simulink model "gm_am_demod_hdl_coder_vnl"  (R2021b)
settings: Solver=FixedStepAuto  StartTime=0.0  StopTime=20  RelTol=1e-3  EnableMultiTasking=on
libraries: hdlmdlgenlib x10, simulink x1
settings Model: Creator=caccolillo  LastModifiedBy=caccolillo
settings SolverCC: AutoInsertRateTranBlk=on
settings OptimizationCC: BlockReduction=off  ConditionallyExecuteInputs=off  DefaultParameterBehavior=Inlined  UseDivisionForNetSlopeComputation=on  GainParamInheritBuiltInType=on  UseFloatMulNetSlope=on  InlineInvariantSignals=on  EfficientFloat2IntCast=on  LifeSpan=1
settings DebuggingCC: AlgebraicLoopMsg=error  InheritedTsInSrcMsg=none  SingleTaskRateTransMsg=error
settings HardwareCC: ProdBitPerPointer=32  ProdBitPerSizeT=32  ProdBitPerPtrDiffT=32  ProdLargestAtomicFloat=None  ProdIntDivRoundTo=Undefined  ProdEndianess=Unspecified  ProdWordSize=32  ProdHWDeviceType=ASIC/FPGA->ASIC/FPGA  TargetBitPerLong=64  TargetBitPerPointer=64  TargetBitPerSizeT=64  TargetBitPerPtrDiffT=64  TargetLongLongMode=on  TargetIntDivRoundTo=Zero  TargetEndianess=LittleEndian  TargetWordSize=64  TargetHWDeviceType=Custom Processor->MATLAB Host Computer  ProdEqTarget=off
settings SFSimCC: MATLABDynamicMemAlloc=off
settings RTWCC: GenerateReport=on  LaunchReport=on
settings CodeAppCC: ForceParamTrailComments=on
settings GRTTargetCC: CombineSignalStateStructs=on  MatFileLogging=off  SupportVariableSizeSignals=on

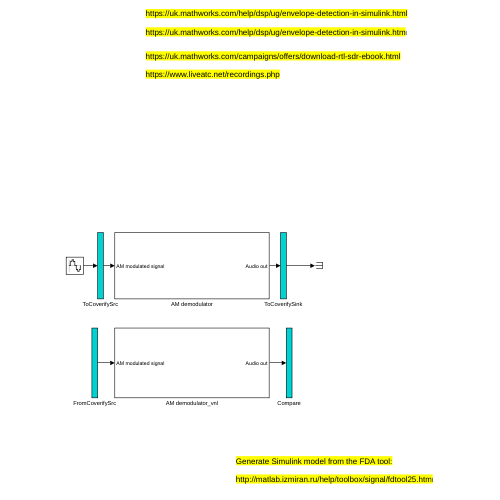
[thumbnail: Simulink's stored preview of the top-level diagram]
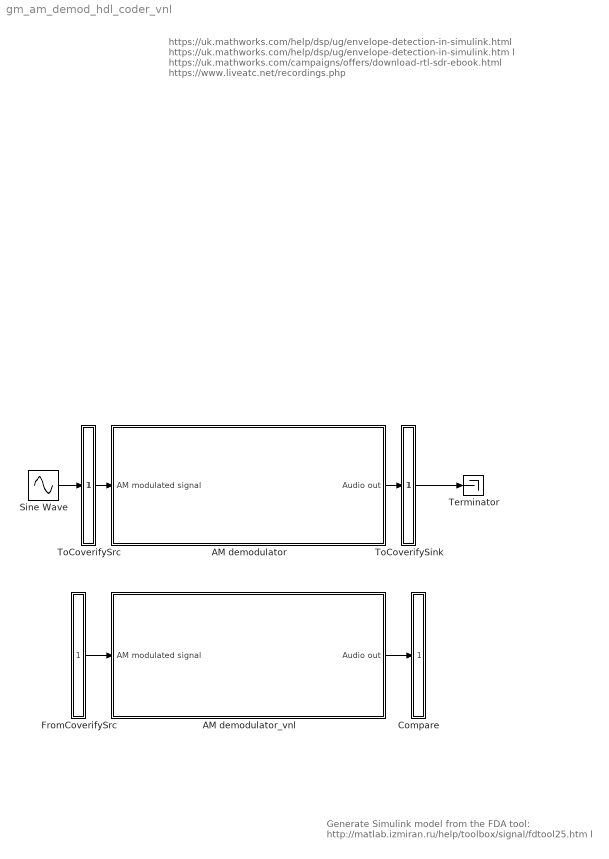
== system gm_am_demod_hdl_coder_vnl ==
  note: Generate Simulink model from the FDA tool:
      |
      | http://matlab.izmiran.ru/help/toolbox/signal/fdtool25.htm l
  note: https://uk.mathworks.com/help/dsp/ug/envelope-detection-in-simulink.html
      |
      | https://uk.mathworks.com/help/dsp/ug/envelope-detection-in-simulink.htm l
      |
      | https://uk.mathworks.com/campaigns/offers/download-rtl-sdr-ebook.html
      |
      | https://www.liveatc.net/recordings.php
  AM demodulator : Subsystem
  AM demodulator_vnl : Subsystem
  Compare : Subsystem
      mask Display: disp('')
  FromCoverifySrc : Subsystem
      mask Display: disp('')
  Sine Wave : Sin  SampleTime=1e-6
  Terminator : Terminator
  ToCoverifySink : Subsystem
      mask Display: disp('')
  ToCoverifySrc : Subsystem
      mask Display: disp('')
  wires:
  ToCoverifySrc/1(out1) -> AM demodulator/1(AM modulated signal)
  AM demodulator/1(Audio out) -> ToCoverifySink/1(in1)
  Sine Wave/1 -> ToCoverifySrc/1(in1)
  ToCoverifySink/1(out1) -> Terminator/1
  FromCoverifySrc/1(out1) -> AM demodulator_vnl/1(AM modulated signal)
  AM demodulator_vnl/1(Audio out) -> Compare/1(in1)

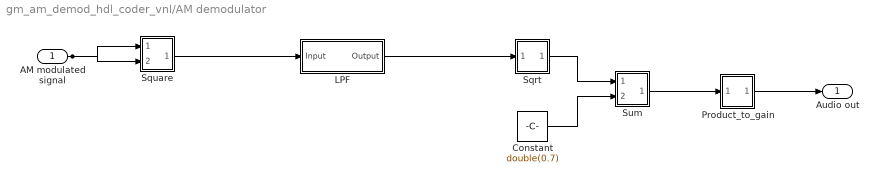
== system gm_am_demod_hdl_coder_vnl/AM demodulator ==
  AM modulated signal : Inport  OutDataTypeStr=double  PortDimensions=1  SampleTime=1e-06
  Constant : Constant  Value=double(0.7)  OutDataTypeStr=double  SampleTime=1e-06
  LPF : Subsystem
  Product_to_gain : Subsystem
      mask Display: disp('NFP\ngain_pow2');
  Sqrt : Subsystem
      mask Display: disp('NFP\nsqrt');
  Square : Subsystem
      mask Display: disp('NFP\nmul');
  Sum : Subsystem
      mask Display: disp('NFP\nadd');
  Audio out : Outport  SampleTime=1e-06
  wires:
  Product_to_gain/1(Out1) -> Audio out/1
  Sum/1(Out1) -> Product_to_gain/1(In1)
  Square/1(Out1) -> LPF/1(Input)
  Sqrt/1(Out1) -> Sum/1(In1)
  LPF/1(Output) -> Sqrt/1(In1)
  Constant/1 -> Sum/2(In2)
  AM modulated signal/1 -> Square/1(In1), Square/2(In2)

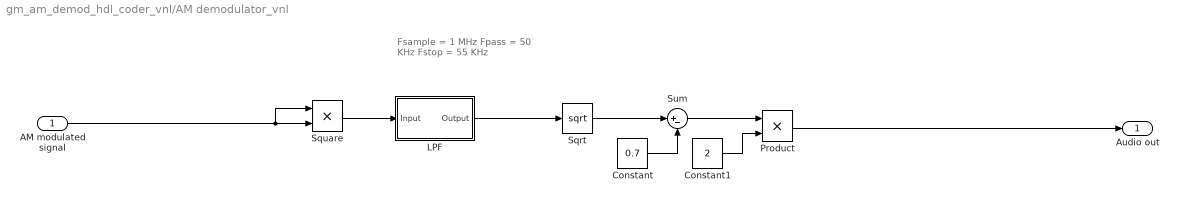
== system gm_am_demod_hdl_coder_vnl/AM demodulator_vnl ==
  note: Fsample = 1 MHz
      | Fpass =  50 KHz
      | Fstop =  55 KHz
  AM modulated signal : Inport  SampleTime=1e-6
  Constant : Constant  Value=0.7  SampleTime=1e-6
  Constant1 : Constant  Value=2  SampleTime=1e-6
  LPF : Subsystem  Tag=FilterWizardSubSystem
      settings: ErrorFcn=dspFilterRealizedInBasicElemsAlgLoopErrFcnCallback
  Product : Product
  Sqrt : Sqrt  SaturateOnIntegerOverflow=on
  Square : Product
  Sum : Sum  Inputs=|+-
  Audio out : Outport
  wires:
  Product/1 -> Audio out/1
  LPF/1(Output) -> Sqrt/1
  Constant1/1 -> Product/2
  Sum/1 -> Product/1
  Constant/1 -> Sum/2
  AM modulated signal/1 -> Square/2, Square/1
  Sqrt/1 -> Sum/1
  Square/1 -> LPF/1(Input)

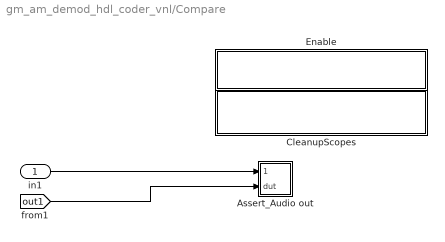
== system gm_am_demod_hdl_coder_vnl/Compare ==
  in1 : Inport
  Assert_Audio out : Subsystem  mask{ToleranceValue=1e-07}
  CleanupScopes : Subsystem
      settings: OpenFcn=|
      | blkName = gcb; %self block
      | idx = regexp(blkName, '/CleanupScopes$', 'once');
      | blkParent = blkName(1:idx-1);
      | blks=find_system(blkParent, 'LookUnderMasks', 'all','blocktype', 'Scope');
      | for itr = 1:length(blks)
      | 	 hScopeCfg = get_param(blks{itr},'ScopeConfiguration');
      | 	 hScopeCfg.Visible = ~ hScopeCfg.Visible;
      | end
      | drawnow;
      mask Display: fprintf(message('hdlcoder:cosim:vnl_dblclick').getString());
  Enable : Subsystem
      settings: OpenFcn=|
      | blkName = gcb;
      | idx = regexp(blkName, '/Enable$', 'once');
      | blkParent = blkName(1:idx-1);
      | blks=find_system(blkParent, 'LookUnderMasks', 'all','blocktype', 'Assertion');
      | e = get_param(blks{1}, 'Enabled');
      | if strcmp(e, 'on'), f= 'off';, else, f = 'on';, end
      | for ii=1:length(blks), set_param(blks{ii}, 'Enabled', f);, end
      | set_param(gcb, 'MaskDisplay',['fprintf(message(''hdlcoder:cosim:vnl_dblclick_assertions'',','''',upper(e),'''',').getString())']);
      mask Display: fprintf(message('hdlcoder:cosim:vnl_dblclick_assertions','OFF').getString());
  wires:
  in1/1 -> Assert_Audio out/1(cosim)
  [out1] -> Assert_Audio out/2(dut)

== system gm_am_demod_hdl_coder_vnl/FromCoverifySrc ==
  out1 : Outport
  wires:
  [in1] -> out1/1

== system gm_am_demod_hdl_coder_vnl/ToCoverifySink ==
  in1 : Inport
  out1 : Outport
  tag scope: out1=global
  wires:
  in1/1 -> out1/1, [out1]

== system gm_am_demod_hdl_coder_vnl/ToCoverifySrc ==
  in1 : Inport
  out1 : Outport
  tag scope: in1=global
  wires:
  in1/1 -> out1/1, [in1]

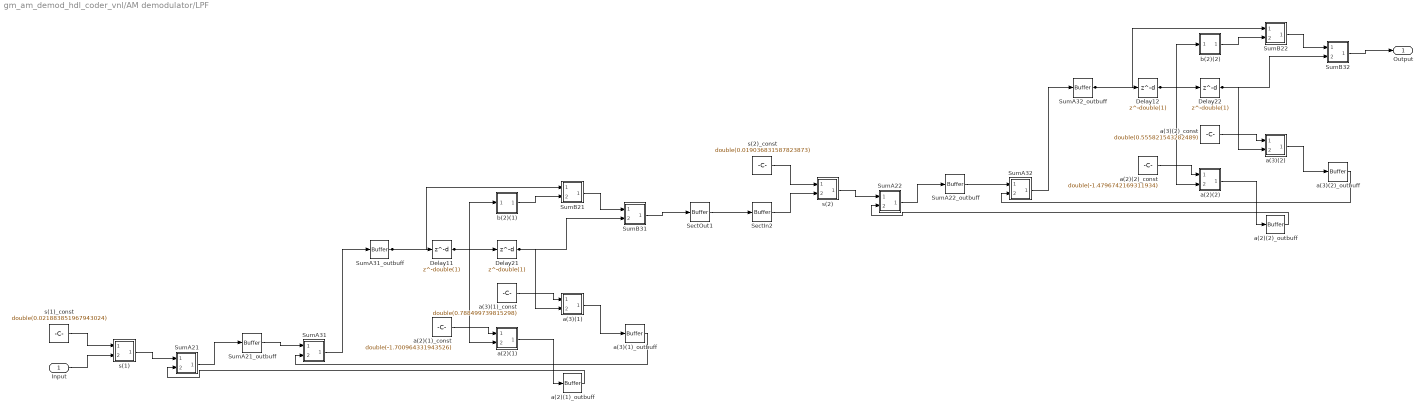
== system gm_am_demod_hdl_coder_vnl/AM demodulator/LPF ==
  Input : Inport  OutDataTypeStr=double  PortDimensions=1  SampleTime=1e-06
  Delay{11..12,21..22} (4 alike) : Delay  DelayLength=double(1)  InitialCondition=0  SampleTime=1e-06
  SectIn2 : hdlmdlgenlib/Buffer
      settings: SourceProductBaseCode=SL
  SectOut1 : hdlmdlgenlib/Buffer
      settings: SourceProductBaseCode=SL
  SumA21 : Subsystem
      mask Display: disp('NFP\nadd');
  SumA21_outbuff : hdlmdlgenlib/Buffer
      settings: SourceProductBaseCode=SL
  SumA22 : Subsystem
      mask Display: disp('NFP\nadd');
  SumA22_outbuff : hdlmdlgenlib/Buffer
      settings: SourceProductBaseCode=SL
  SumA31 : Subsystem
      mask Display: disp('NFP\nadd');
  SumA31_outbuff : hdlmdlgenlib/Buffer
      settings: SourceProductBaseCode=SL
  SumA32 : Subsystem
      mask Display: disp('NFP\nadd');
  SumA32_outbuff : hdlmdlgenlib/Buffer
      settings: SourceProductBaseCode=SL
  SumB21 : Subsystem
      mask Display: disp('NFP\nadd');
  SumB22 : Subsystem
      mask Display: disp('NFP\nadd');
  SumB31 : Subsystem
      mask Display: disp('NFP\nadd');
  SumB32 : Subsystem
      mask Display: disp('NFP\nadd');
  a(2)(1) : Subsystem
      mask Display: disp('NFP\nmul');
  a(2)(1)_const : Constant  Value=double(-1.700964331943526)  OutDataTypeStr=double  SampleTime=1e-06
  a(2)(1)_outbuff : hdlmdlgenlib/Buffer
      settings: SourceProductBaseCode=SL
  a(2)(2) : Subsystem
      mask Display: disp('NFP\nmul');
  a(2)(2)_const : Constant  Value=double(-1.4796742169311934)  OutDataTypeStr=double  SampleTime=1e-06
  a(2)(2)_outbuff : hdlmdlgenlib/Buffer
      settings: SourceProductBaseCode=SL
  a(3)(1) : Subsystem
      mask Display: disp('NFP\nmul');
  a(3)(1)_const : Constant  Value=double(0.788499739815298)  OutDataTypeStr=double  SampleTime=1e-06
  a(3)(1)_outbuff : hdlmdlgenlib/Buffer
      settings: SourceProductBaseCode=SL
  a(3)(2) : Subsystem
      mask Display: disp('NFP\nmul');
  a(3)(2)_const : Constant  Value=double(0.555821543282489)  OutDataTypeStr=double  SampleTime=1e-06
  a(3)(2)_outbuff : hdlmdlgenlib/Buffer
      settings: SourceProductBaseCode=SL
  b(2)(1) : Subsystem
      mask Display: disp('NFP\ngain_pow2');
  b(2)(2) : Subsystem
      mask Display: disp('NFP\ngain_pow2');
  s(1) : Subsystem
      mask Display: disp('NFP\nmul');
  s(1)_const : Constant  Value=double(0.021883851967943024)  OutDataTypeStr=double  SampleTime=1e-06
  s(2) : Subsystem
      mask Display: disp('NFP\nmul');
  s(2)_const : Constant  Value=double(0.019036831587823873)  OutDataTypeStr=double  SampleTime=1e-06
  Output : Outport  SampleTime=1e-06
  wires:
  s(2)/1(Out1) -> SumA22/1(In1)
  s(1)/1(Out1) -> SumA21/1(In1)
  a(3)(2)/1(Out1) -> a(3)(2)_outbuff/1
  a(3)(1)/1(Out1) -> a(3)(1)_outbuff/1
  a(2)(2)/1(Out1) -> a(2)(2)_outbuff/1
  a(2)(1)/1(Out1) -> a(2)(1)_outbuff/1
  SumB32/1(Out1) -> Output/1
  SumB31/1(Out1) -> SectOut1/1
  SumB22/1(Out1) -> SumB32/1(In1)
  SumB21/1(Out1) -> SumB31/1(In1)
  SumA32/1(Out1) -> SumA32_outbuff/1
  SumA31/1(Out1) -> SumA31_outbuff/1
  SumA22/1(Out1) -> SumA22_outbuff/1
  SumA21/1(Out1) -> SumA21_outbuff/1
  b(2)(2)/1(Out1) -> SumB22/2(In2)
  b(2)(1)/1(Out1) -> SumB21/2(In2)
  s(2)_const/1 -> s(2)/1(In1)
  s(1)_const/1 -> s(1)/1(In1)
  a(3)(2)_const/1 -> a(3)(2)/1(In1)
  a(3)(1)_const/1 -> a(3)(1)/1(In1)
  a(2)(2)_const/1 -> a(2)(2)/1(In1)
  a(2)(1)_const/1 -> a(2)(1)/1(In1)
  SectOut1/1 -> SectIn2/1
  a(3)(2)_outbuff/1 -> SumA32/2(In2)
  a(3)(1)_outbuff/1 -> SumA31/2(In2)
  a(2)(2)_outbuff/1 -> SumA22/2(In2)
  a(2)(1)_outbuff/1 -> SumA21/2(In2)
  SumA32_outbuff/1 -> Delay12/1, SumB22/1(In1)
  SumA31_outbuff/1 -> Delay11/1, SumB21/1(In1)
  SumA22_outbuff/1 -> SumA32/1(In1)
  SumA21_outbuff/1 -> SumA31/1(In1)
  SectIn2/1 -> s(2)/2(In2)
  Delay22/1 -> SumB32/2(In2), a(3)(2)/2(In2)
  Delay21/1 -> SumB31/2(In2), a(3)(1)/2(In2)
  Delay12/1 -> Delay22/1, b(2)(2)/1(In1), a(2)(2)/2(In2)
  Delay11/1 -> Delay21/1, b(2)(1)/1(In1), a(2)(1)/2(In2)
  Input/1 -> s(1)/2(In2)

== system gm_am_demod_hdl_coder_vnl/AM demodulator/Product_to_gain ==
  In1 : Inport
  Product_to_gain : Gain  Gain=double(2)
  Out1 : Outport
  wires:
  Product_to_gain/1 -> Out1/1
  In1/1 -> Product_to_gain/1

== system gm_am_demod_hdl_coder_vnl/AM demodulator/Sqrt ==
  In1 : Inport
  Sqrt : Sqrt  SampleTime=1e-06  SaturateOnIntegerOverflow=on
  Out1 : Outport
  wires:
  Sqrt/1 -> Out1/1
  In1/1 -> Sqrt/1

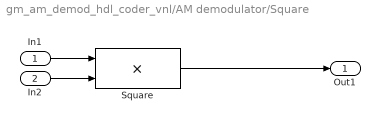
== system gm_am_demod_hdl_coder_vnl/AM demodulator/Square ==
  In1 : Inport
  In2 : Inport  Port=2
  Square : Product  Inputs=**  OutDataTypeStr=double  SampleTime=1e-06
  Out1 : Outport
  wires:
  Square/1 -> Out1/1
  In2/1 -> Square/2
  In1/1 -> Square/1

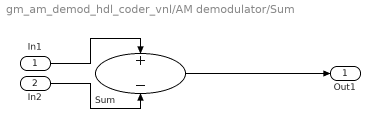
== system gm_am_demod_hdl_coder_vnl/AM demodulator/Sum ==
  In1 : Inport
  In2 : Inport  Port=2
  Sum : Sum  Inputs=+-  OutDataTypeStr=double  SampleTime=1e-06
  Out1 : Outport
  wires:
  Sum/1 -> Out1/1
  In2/1 -> Sum/2
  In1/1 -> Sum/1

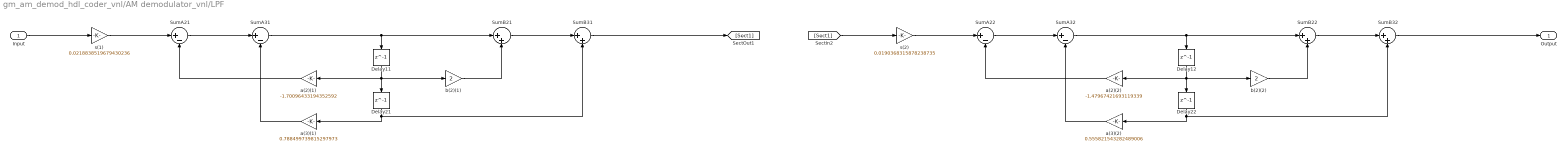
== system gm_am_demod_hdl_coder_vnl/AM demodulator_vnl/LPF ==
  Input : Inport
  Delay{11..12,21..22} (4 alike) : Delay  DelayLength=1  InitialCondition=0
  SumA{21..22,31..32} (4 alike) : Sum  Inputs=|+-  RndMeth=Nearest  SaturateOnIntegerOverflow=on  OutDataTypeStr=Inherit: Same as first input
  SumB{21..22,31..32} (4 alike) : Sum  Inputs=|++  RndMeth=Nearest  SaturateOnIntegerOverflow=on  OutDataTypeStr=Inherit: Same as first input
  a(2)(1) : Gain  Gain=-1.70096433194352592  ParamDataTypeStr=double  RndMeth=Nearest  SaturateOnIntegerOverflow=on  OutDataTypeStr=Inherit: Same as input
  a(2)(2) : Gain  Gain=-1.47967421693119339  ParamDataTypeStr=double  RndMeth=Nearest  SaturateOnIntegerOverflow=on  OutDataTypeStr=Inherit: Same as input
  a(3)(1) : Gain  Gain=0.788499739815297973  ParamDataTypeStr=double  RndMeth=Nearest  SaturateOnIntegerOverflow=on  OutDataTypeStr=Inherit: Same as input
  a(3)(2) : Gain  Gain=0.555821543282489006  ParamDataTypeStr=double  RndMeth=Nearest  SaturateOnIntegerOverflow=on  OutDataTypeStr=Inherit: Same as input
  b(2)(1) : Gain  Gain=2  ParamDataTypeStr=double  RndMeth=Nearest  SaturateOnIntegerOverflow=on  OutDataTypeStr=Inherit: Same as input
  b(2)(2) : Gain  Gain=2  ParamDataTypeStr=double  RndMeth=Nearest  SaturateOnIntegerOverflow=on  OutDataTypeStr=Inherit: Same as input
  s(1) : Gain  Gain=0.0218838519679430236  ParamDataTypeStr=double  RndMeth=Nearest  SaturateOnIntegerOverflow=on  OutDataTypeStr=Inherit: Same as input
  s(2) : Gain  Gain=0.0190368315878238735  ParamDataTypeStr=double  RndMeth=Nearest  SaturateOnIntegerOverflow=on  OutDataTypeStr=Inherit: Same as input
  Output : Outport
  wires:
  Delay22/1 -> SumB32/2, a(3)(2)/1
  a(3)(2)/1 -> SumA32/2
  b(2)(2)/1 -> SumB22/2
  Delay12/1 -> Delay22/1, b(2)(2)/1, a(2)(2)/1
  a(2)(2)/1 -> SumA22/2
  SumB32/1 -> Output/1
  SumB22/1 -> SumB32/1
  SumA32/1 -> Delay12/1, SumB22/1
  SumA22/1 -> SumA32/1
  s(2)/1 -> SumA22/1
  [Sect1] -> s(2)/1
  Delay21/1 -> SumB31/2, a(3)(1)/1
  a(3)(1)/1 -> SumA31/2
  b(2)(1)/1 -> SumB21/2
  Delay11/1 -> Delay21/1, b(2)(1)/1, a(2)(1)/1
  a(2)(1)/1 -> SumA21/2
  SumB31/1 -> [Sect1]
  SumB21/1 -> SumB31/1
  SumA31/1 -> Delay11/1, SumB21/1
  SumA21/1 -> SumA31/1
  s(1)/1 -> SumA21/1
  Input/1 -> s(1)/1

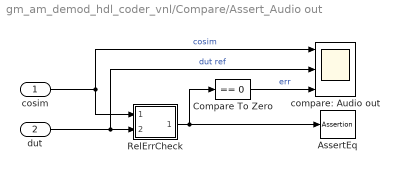
== system gm_am_demod_hdl_coder_vnl/Compare/Assert_Audio out ==
  cosim : Inport
  dut : Inport  Port=2
  AssertEq : Assertion  StopWhenAssertionFail=off
  Compare To Zero : simulink/Logic and Bit Operations/Compare To Zero  relop===  OutDataTypeStr=boolean
  RelErrCheck : Subsystem
  compare: Audio out : Scope  NumInputPorts=3
  wires:
  dut/1 -> compare: Audio out/2, RelErrCheck/2(In2)  "dut ref"
  cosim/1 -> compare: Audio out/1, RelErrCheck/1(In1)  "cosim"
  RelErrCheck/1(Out1) -> AssertEq/1, Compare To Zero/1
  Compare To Zero/1 -> compare: Audio out/3  "err"

== system gm_am_demod_hdl_coder_vnl/Compare/CleanupScopes ==

== system gm_am_demod_hdl_coder_vnl/Compare/Enable ==

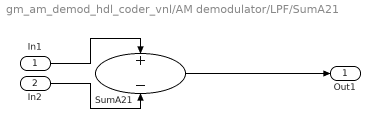
== system gm_am_demod_hdl_coder_vnl/AM demodulator/LPF/SumA21 ==
  In1 : Inport
  In2 : Inport  Port=2
  SumA21 : Sum  Inputs=+-  OutDataTypeStr=double  RndMeth=Nearest  SampleTime=1e-06
  Out1 : Outport
  wires:
  SumA21/1 -> Out1/1
  In2/1 -> SumA21/2
  In1/1 -> SumA21/1

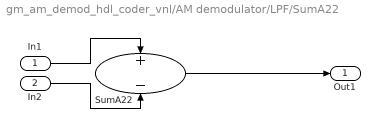
== system gm_am_demod_hdl_coder_vnl/AM demodulator/LPF/SumA22 ==
  In1 : Inport
  In2 : Inport  Port=2
  SumA22 : Sum  Inputs=+-  OutDataTypeStr=double  RndMeth=Nearest  SampleTime=1e-06
  Out1 : Outport
  wires:
  SumA22/1 -> Out1/1
  In2/1 -> SumA22/2
  In1/1 -> SumA22/1

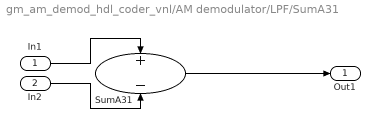
== system gm_am_demod_hdl_coder_vnl/AM demodulator/LPF/SumA31 ==
  In1 : Inport
  In2 : Inport  Port=2
  SumA31 : Sum  Inputs=+-  OutDataTypeStr=double  RndMeth=Nearest  SampleTime=1e-06
  Out1 : Outport
  wires:
  SumA31/1 -> Out1/1
  In2/1 -> SumA31/2
  In1/1 -> SumA31/1

== system gm_am_demod_hdl_coder_vnl/AM demodulator/LPF/SumA32 ==
  In1 : Inport
  In2 : Inport  Port=2
  SumA32 : Sum  Inputs=+-  OutDataTypeStr=double  RndMeth=Nearest  SampleTime=1e-06
  Out1 : Outport
  wires:
  SumA32/1 -> Out1/1
  In2/1 -> SumA32/2
  In1/1 -> SumA32/1

== system gm_am_demod_hdl_coder_vnl/AM demodulator/LPF/SumB21 ==
  In1 : Inport
  In2 : Inport  Port=2
  SumB21 : Sum  OutDataTypeStr=double  RndMeth=Nearest  SampleTime=1e-06
  Out1 : Outport
  wires:
  SumB21/1 -> Out1/1
  In2/1 -> SumB21/2
  In1/1 -> SumB21/1

== system gm_am_demod_hdl_coder_vnl/AM demodulator/LPF/SumB22 ==
  In1 : Inport
  In2 : Inport  Port=2
  SumB22 : Sum  OutDataTypeStr=double  RndMeth=Nearest  SampleTime=1e-06
  Out1 : Outport
  wires:
  SumB22/1 -> Out1/1
  In2/1 -> SumB22/2
  In1/1 -> SumB22/1

== system gm_am_demod_hdl_coder_vnl/AM demodulator/LPF/SumB31 ==
  In1 : Inport
  In2 : Inport  Port=2
  SumB31 : Sum  OutDataTypeStr=double  RndMeth=Nearest  SampleTime=1e-06
  Out1 : Outport
  wires:
  SumB31/1 -> Out1/1
  In2/1 -> SumB31/2
  In1/1 -> SumB31/1

== system gm_am_demod_hdl_coder_vnl/AM demodulator/LPF/SumB32 ==
  In1 : Inport
  In2 : Inport  Port=2
  SumB32 : Sum  OutDataTypeStr=double  RndMeth=Nearest  SampleTime=1e-06
  Out1 : Outport
  wires:
  SumB32/1 -> Out1/1
  In2/1 -> SumB32/2
  In1/1 -> SumB32/1

== system gm_am_demod_hdl_coder_vnl/AM demodulator/LPF/a(2)(1) ==
  In1 : Inport
  In2 : Inport  Port=2
  a(2)(1) : Product  Inputs=**  OutDataTypeStr=double  RndMeth=Nearest  SaturateOnIntegerOverflow=on  SampleTime=1e-06
  Out1 : Outport
  wires:
  a(2)(1)/1 -> Out1/1
  In2/1 -> a(2)(1)/2
  In1/1 -> a(2)(1)/1

== system gm_am_demod_hdl_coder_vnl/AM demodulator/LPF/a(2)(2) ==
  In1 : Inport
  In2 : Inport  Port=2
  a(2)(2) : Product  Inputs=**  OutDataTypeStr=double  RndMeth=Nearest  SaturateOnIntegerOverflow=on  SampleTime=1e-06
  Out1 : Outport
  wires:
  a(2)(2)/1 -> Out1/1
  In2/1 -> a(2)(2)/2
  In1/1 -> a(2)(2)/1

== system gm_am_demod_hdl_coder_vnl/AM demodulator/LPF/a(3)(1) ==
  In1 : Inport
  In2 : Inport  Port=2
  a(3)(1) : Product  Inputs=**  OutDataTypeStr=double  RndMeth=Nearest  SaturateOnIntegerOverflow=on  SampleTime=1e-06
  Out1 : Outport
  wires:
  a(3)(1)/1 -> Out1/1
  In2/1 -> a(3)(1)/2
  In1/1 -> a(3)(1)/1

== system gm_am_demod_hdl_coder_vnl/AM demodulator/LPF/a(3)(2) ==
  In1 : Inport
  In2 : Inport  Port=2
  a(3)(2) : Product  Inputs=**  OutDataTypeStr=double  RndMeth=Nearest  SaturateOnIntegerOverflow=on  SampleTime=1e-06
  Out1 : Outport
  wires:
  a(3)(2)/1 -> Out1/1
  In2/1 -> a(3)(2)/2
  In1/1 -> a(3)(2)/1

== system gm_am_demod_hdl_coder_vnl/AM demodulator/LPF/b(2)(1) ==
  In1 : Inport
  b(2)(1) : Gain  Gain=double(2)  RndMeth=Nearest  SaturateOnIntegerOverflow=on
  Out1 : Outport
  wires:
  b(2)(1)/1 -> Out1/1
  In1/1 -> b(2)(1)/1

== system gm_am_demod_hdl_coder_vnl/AM demodulator/LPF/b(2)(2) ==
  In1 : Inport
  b(2)(2) : Gain  Gain=double(2)  RndMeth=Nearest  SaturateOnIntegerOverflow=on
  Out1 : Outport
  wires:
  b(2)(2)/1 -> Out1/1
  In1/1 -> b(2)(2)/1

== system gm_am_demod_hdl_coder_vnl/AM demodulator/LPF/s(1) ==
  In1 : Inport
  In2 : Inport  Port=2
  s(1) : Product  Inputs=**  OutDataTypeStr=double  RndMeth=Nearest  SaturateOnIntegerOverflow=on  SampleTime=1e-06
  Out1 : Outport
  wires:
  s(1)/1 -> Out1/1
  In2/1 -> s(1)/2
  In1/1 -> s(1)/1

== system gm_am_demod_hdl_coder_vnl/AM demodulator/LPF/s(2) ==
  In1 : Inport
  In2 : Inport  Port=2
  s(2) : Product  Inputs=**  OutDataTypeStr=double  RndMeth=Nearest  SaturateOnIntegerOverflow=on  SampleTime=1e-06
  Out1 : Outport
  wires:
  s(2)/1 -> Out1/1
  In2/1 -> s(2)/2
  In1/1 -> s(2)/1

== system gm_am_demod_hdl_coder_vnl/Compare/Assert_Audio out/RelErrCheck ==
  In1 : Inport
  In2 : Inport  Port=2
  "RelativeErrorCheck " : MATLAB Function  TreatAsAtomicUnit=on
  Out1 : Outport  VectorParamsAs1DForOutWhenUnconnected=off
  wires:
  In2/1 -> "RelativeErrorCheck "/2(R)
  In1/1 -> "RelativeErrorCheck "/1(P)
  "RelativeErrorCheck "/1(y) -> Out1/1

== matlab function gm_am_demod_hdl_coder_vnl/Compare/Assert_Audio out/RelErrCheck/RelativeErrorCheck  ==
  data: P input; y output; R input; ToleranceValue parameter double
% Check if the relative error of R with respect to P is below
% ToleranceValue
% P, R are floating-point
function y = relErrCheck(P,R, ToleranceValue)
    tol = ToleranceValue;
    sz = numel(P);
    assert(sz == numel(R), 'Inputs P and R have different sizes.');
    y = false(1, sz);

    for ii=1:sz
        if (isnan(P(ii)) || isnan(R(ii)))
            if (isnan(P(ii)) && isnan(R(ii)))
                y(ii) = true;
            end
        elseif (isinf(P(ii)) || isinf(R(ii)))
            y(ii) = (P(ii) == R(ii));
        elseif (P(ii) == 0)
            y(ii) = (R(ii) == 0);
        else
            absdiff = abs(P(ii) - R(ii));
            relerr = absdiff/abs(P(ii));
            y(ii) = (relerr <= tol);
        end
    end
end
